simulink model "Straight_line"  (R2021a)
settings: Solver=VariableStepAuto  StartTime=0.0  StopTime=60  RelTol=1e-3  AbsTol=1e-3  EnableMultiTasking=on
values from neighbouring files (symbols this model uses):
  m = rho * V    [Tinh_I_va_m.m]
libraries: sm_lib x11, nesl_utility x10, simulink x5
settings Model: Creator=Administrator  LastModifiedBy=Administrator
settings SolverCC: AutoScaleAbsTol=off  ZeroCrossAlgorithm=Adaptive  AlgebraicLoopSolver=TrustRegion
settings DataIOCC: LimitDataPoints=on  MaxDataPoints=10000
settings OptimizationCC: LifeSpan=inf
settings DebuggingCC: IgnoredZcDiagnostic=none  AllowSymbolicDim=off  SFUnexpectedBacktrackingDiag=warning  SFNoUnconditionalDefaultTransitionDiag=warning  SFExecutionAtInitializationDiag=none  SFMachineParentedDataDiag=warning  ArithmeticOperatorsInVariantConditions=warning
settings SFSimCC: SimUseLocalCustomCode=off  CustomCodeUndefinedFunction=UseInterfaceOnly
settings RTWCC: RTWUseLocalCustomCode=off
settings CodeAppCC: StateflowObjectComments=on
settings GRTTargetCC: TargetLangStandard=C89/C90 (ANSI)
settings ConfigComp: CovMetricSettings=dw  CovSaveCumulativeToWorkspaceVar=on  CovSaveSingleToWorkspaceVar=on  CovExternalEMLEnable=off  CovSFcnEnable=off
settings SimscapeCC: SimscapeLogType=all  SimscapeLogSimulationStatistics=on  SimscapeLogDataHistory=10000

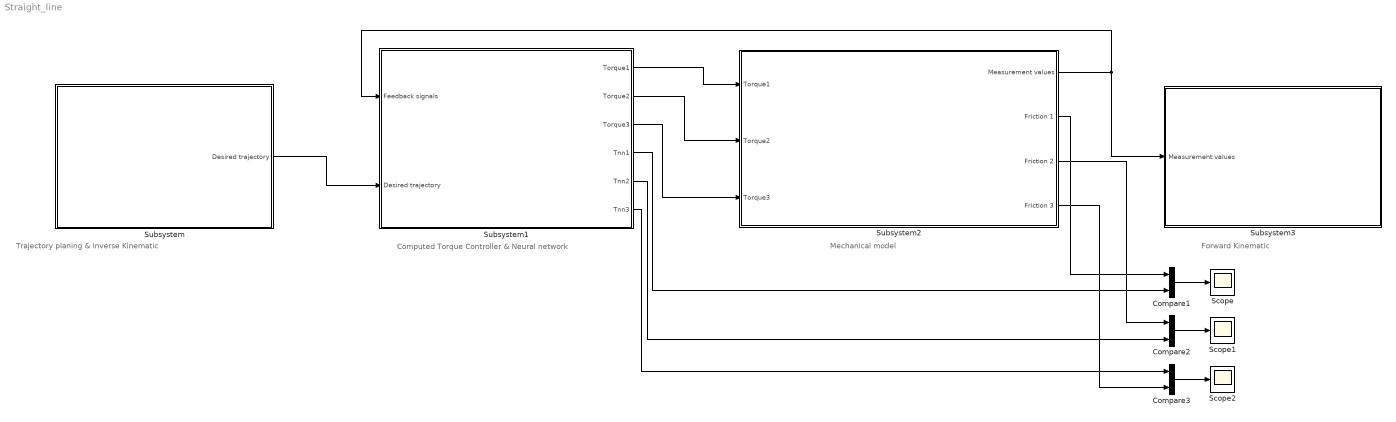
== system Straight_line ==
  note: Trajectory planing & Inverse Kinematic
  note: Computed Torque Controller
      | & Neural network
  note: Mechanical model
  note: Forward Kinematic
  Compare1 : Mux  Inputs=2
  Compare2 : Mux  Inputs=2
  Compare3 : Mux  Inputs=2
  Scope : Scope
  Scope1 : Scope
  Scope2 : Scope
  Subsystem : Subsystem
  Subsystem1 : Subsystem
  Subsystem2 : Subsystem
  Subsystem3 : Subsystem
  wires:
  Subsystem/1("Desired trajectory ") -> Subsystem1/2(Desired trajectory)
  Subsystem1/1(Torque1) -> Subsystem2/1(Torque1)
  Subsystem2/1(Measurement values) -> Subsystem1/1(Feedback signals), Subsystem3/1(Measurement values)
  Subsystem1/2(Torque2) -> Subsystem2/2(Torque2)
  Subsystem1/3(Torque3) -> Subsystem2/3(Torque3)
  Subsystem2/4(Friction 3) -> Compare3/2
  Subsystem1/6(Tnn3) -> Compare3/1
  Subsystem1/5(Tnn2) -> Compare2/2
  Subsystem2/3(Friction 2) -> Compare2/1
  Subsystem1/4(Tnn1) -> Compare1/2
  Subsystem2/2(Friction 1) -> Compare1/1
  Compare1/1 -> Scope/1
  Compare2/1 -> Scope1/1
  Compare3/1 -> Scope2/1

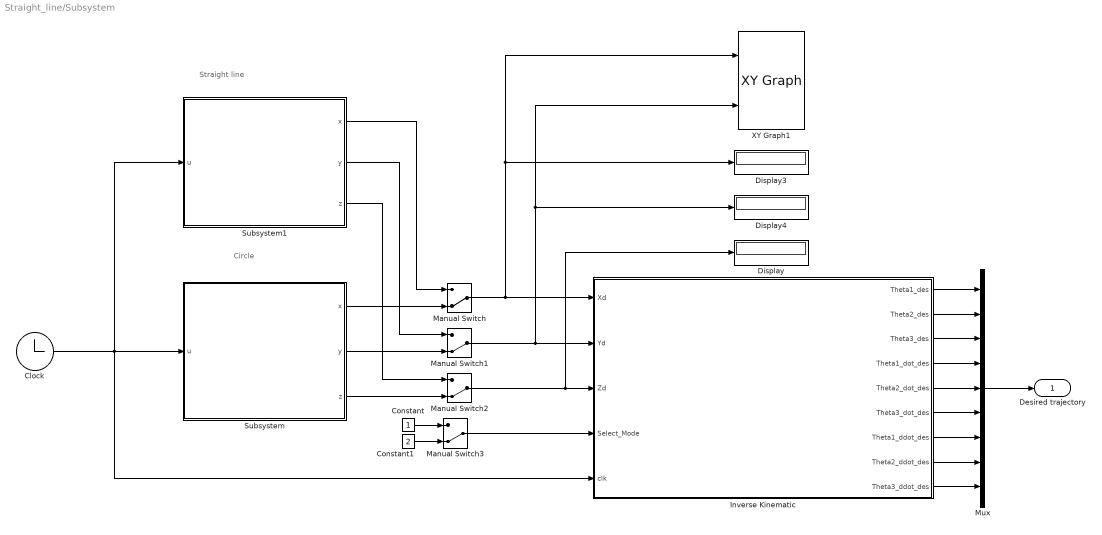
== system Straight_line/Subsystem ==
  note: Circle
  note: Straight line
  Clock : Clock
  Constant : Constant
  Constant1 : Constant  Value=2
  Display : Display
  Display3 : Display
  Display4 : Display
  Inverse Kinematic : MATLAB Function  TreatAsAtomicUnit=on
  Manual Switch{,1..3} (4 alike) : ManualSwitch  CurrentSetting=0
  Mux : Mux  Inputs=9
  Subsystem : Subsystem
  Subsystem1 : Subsystem
  XY Graph1 : simulink/Sinks/XY Graph  xmin=-3  xmax=3  ymin=-3  ymax=3  st=-1
  "Desired trajectory " : Outport
  wires:
  Clock/1 -> Subsystem1/1(u), Inverse Kinematic/5(clk), Subsystem/1(u)
  Inverse Kinematic/1(Theta1_des) -> Mux/1
  Inverse Kinematic/2(Theta2_des) -> Mux/2
  Inverse Kinematic/3(Theta3_des) -> Mux/3
  Inverse Kinematic/4(Theta1_dot_des) -> Mux/4
  Inverse Kinematic/5(Theta2_dot_des) -> Mux/5
  Inverse Kinematic/6(Theta3_dot_des) -> Mux/6
  Inverse Kinematic/7(Theta1_ddot_des) -> Mux/7
  Inverse Kinematic/8(Theta2_ddot_des) -> Mux/8
  Inverse Kinematic/9(Theta3_ddot_des) -> Mux/9
  Subsystem/1(x) -> Manual Switch/2
  Manual Switch/1 -> Inverse Kinematic/1(Xd), XY Graph1/1, Display3/1
  Manual Switch1/1 -> Inverse Kinematic/2(Yd), XY Graph1/2, Display4/1
  Subsystem/2(y) -> Manual Switch1/2
  Manual Switch2/1 -> Inverse Kinematic/3(Zd), Display/1
  Subsystem/3(z) -> Manual Switch2/2
  Mux/1 -> "Desired trajectory "/1
  Subsystem1/1(x) -> Manual Switch/1
  Subsystem1/2(y) -> Manual Switch1/1
  Subsystem1/3(z) -> Manual Switch2/1
  Manual Switch3/1 -> Inverse Kinematic/4(Select_Mode)
  Constant/1 -> Manual Switch3/1
  Constant1/1 -> Manual Switch3/2

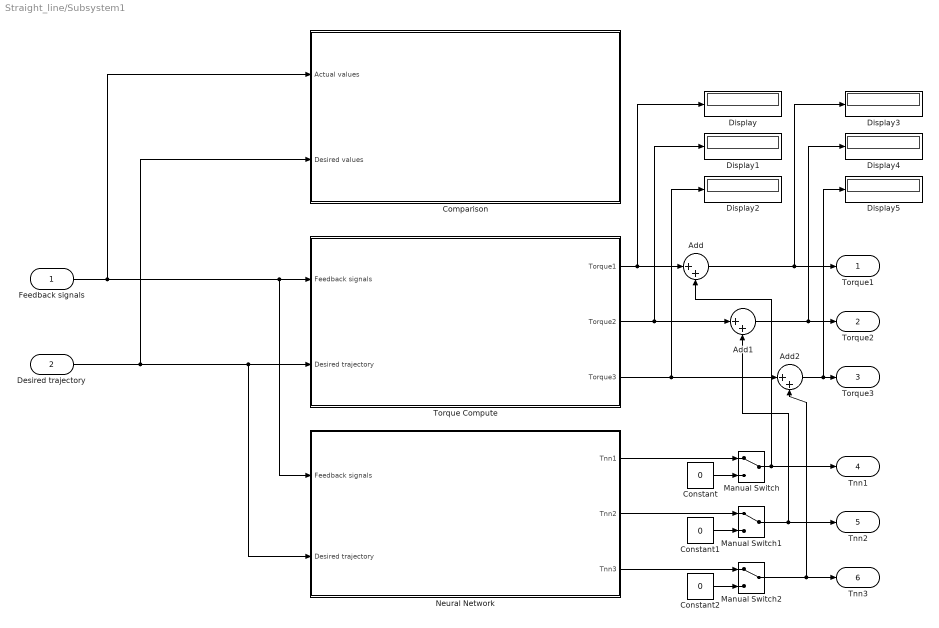
== system Straight_line/Subsystem1 ==
  Feedback signals : Inport
  Desired trajectory : Inport  Port=2
  Add : Sum  Inputs=|++
  Add1 : Sum  Inputs=|++
  Add2 : Sum  Inputs=|++
  Comparison : Subsystem
  Constant : Constant  Value=0
  Constant1 : Constant  Value=0
  Constant2 : Constant  Value=0
  Display{,1..5} (6 alike) : Display
  Manual Switch : ManualSwitch
  Manual Switch1 : ManualSwitch
  Manual Switch2 : ManualSwitch
  Neural Network : Subsystem
  Torque Compute : Subsystem
  Torque1 : Outport
  Torque2 : Outport  Port=2
  Torque3 : Outport  Port=3
  Tnn1 : Outport  Port=4
  Tnn2 : Outport  Port=5
  Tnn3 : Outport  Port=6
  wires:
  Feedback signals/1 -> Comparison/1(Actual values), Neural Network/1(Feedback signals), Torque Compute/1(Feedback signals)
  Desired trajectory/1 -> Comparison/2(Desired values), Torque Compute/2(Desired trajectory), Neural Network/2(Desired trajectory)
  Torque Compute/1(Torque1) -> Display/1, Add/1
  Torque Compute/3(Torque3) -> Display2/1, Add2/1
  Add2/1 -> Display5/1, Torque3/1
  Torque Compute/2(Torque2) -> Display1/1, Add1/1
  Add1/1 -> Display4/1, Torque2/1
  Add/1 -> Display3/1, Torque1/1
  Manual Switch/1 -> Tnn1/1, Add/2
  Constant/1 -> Manual Switch/2
  Constant2/1 -> Manual Switch2/2
  Constant1/1 -> Manual Switch1/2
  Manual Switch1/1 -> Tnn2/1, Add1/2
  Manual Switch2/1 -> Tnn3/1, Add2/2
  Neural Network/3(Tnn3) -> Manual Switch2/1
  Neural Network/2(Tnn2) -> Manual Switch1/1
  Neural Network/1(Tnn1) -> Manual Switch/1

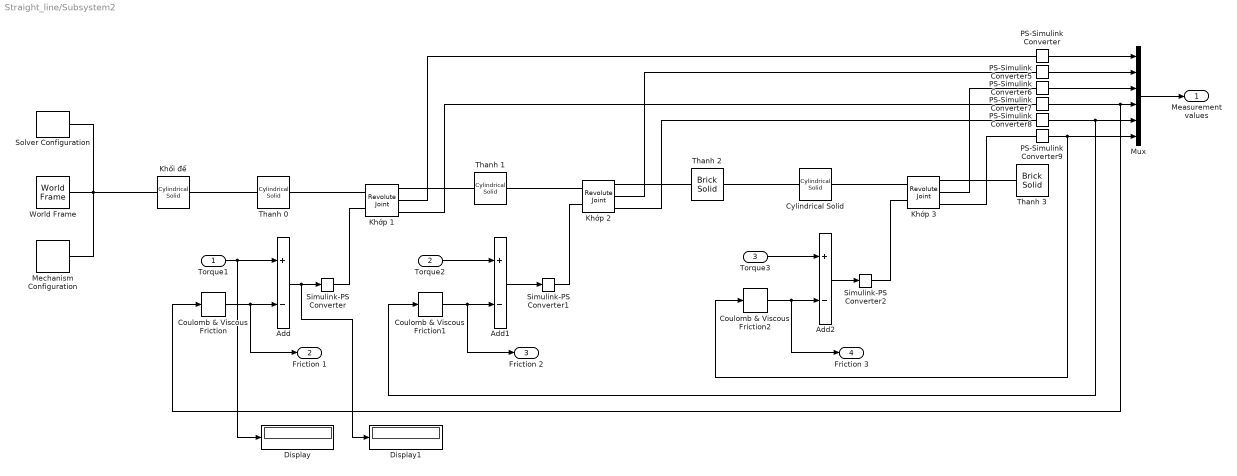
== system Straight_line/Subsystem2 ==
  Torque1 : Inport
  Torque2 : Inport  Port=2
  Torque3 : Inport  Port=3
  Add : Sum  Inputs=+-
  Add1 : Sum  Inputs=+-
  Add2 : Sum  Inputs=+-
  Coulomb & Viscous Friction : simulink/Discontinuities/Coulomb & Viscous Friction  offset=0  gain=0
  Coulomb & Viscous Friction1 : simulink/Discontinuities/Coulomb & Viscous Friction  offset=0  gain=0
  Coulomb & Viscous Friction2 : simulink/Discontinuities/Coulomb & Viscous Friction  offset=0  gain=0
  Cylindrical Solid : sm_lib/Body Elements/Cylindrical Solid  GraphicAmbientColor=[0.15 0.15 0.15 1.0]  BasedOnType=Density  CenterOfMass=[0 0 0]  CenterOfMassUnits=m  GraphicDiffuseColor=[0.8 0.4 1.0]  CylinderLength=0.5  CylinderLengthUnits=m  CylinderRadius=0.5  CylinderRadiusUnits=m  Density=900  DensityUnits=kg/m^3  DoExposeReferenceFrame=off  GraphicEmissiveColor=[0.0 0.0 0.0 1.0]  ExportEntireGeometry=off  SerializedFrames=<Frames><Frame><Id>Frame1</Id><Value><Name>F1</Name><Origin><Source>GeometricFeature</Source><FeatureName>top surface</FeatureName></Origin><PrimaryAxis><DefinedDirection>+Z</DefinedDirection><Source>ReferenceFrame</Source><SourceDirection>+Z</SourceDirection><FeatureName></FeatureName></PrimaryAxis><SecondaryAxis><DefinedDirection>+X</DefinedDirection><Source>ReferenceFrame</Source><SourceDirection>+X</SourceDirection><FeatureName></FeatureName></SecondaryAxis></Value></Frame><Frame><Id>Frame2</Id><Value><Name>F2</Name><Origin><Source>GeometricFeature</Source><FeatureName>bottom surface</FeatureName></Origin><PrimaryAxis><DefinedDirection>+Z</DefinedDirection><Source>ReferenceFrame</Source><SourceDirection>+Z</SourceDirection><FeatureName></FeatureName></PrimaryAxis><SecondaryAxis><DefinedDirection>+X</DefinedDirection><Source>ReferenceFrame</Source><SourceDirection>+X</SourceDirection><FeatureName></FeatureName></SecondaryAxis></Value></Frame></Frames>  MarkerShape=Sphere  MarkerSize=10  GraphicType=FromGeometry  InertiaType=CalculateFromGeometry  Mass=1  MassUnits=kg  MomentsOfInertia=[1 1 1]  MomentsOfInertiaUnits=kg*m^2  GraphicOpacity=1.0  ProductsOfInertia=[0 0 0]  ProductsOfInertiaUnits=kg*m^2  GraphicShininess=75  GraphicSpecularColor=[0.5 0.5 0.5 1.0]  GraphicVisPropType=SimpleVisualProperties
  Display : Display
  Display1 : Display
  Khối đế : sm_lib/Body Elements/Cylindrical Solid  GraphicAmbientColor=[0.15 0.15 0.15 1.0]  BasedOnType=Density  CenterOfMass=[0 0 0]  CenterOfMassUnits=m  GraphicDiffuseColor=[0.2 1.0 0.2]  CylinderLength=8  CylinderLengthUnits=m  CylinderRadius=3  CylinderRadiusUnits=m  Density=900  DensityUnits=kg/m^3  DoExposeReferenceFrame=on  GraphicEmissiveColor=[0.0 0.0 0.0 1.0]  ExportEntireGeometry=off  SerializedFrames=<Frames><Frame><Id>Frame1</Id><Value><Name>Top</Name><Origin><Source>GeometricFeature</Source><FeatureName>top surface</FeatureName></Origin><PrimaryAxis><DefinedDirection>+Z</DefinedDirection><Source>ReferenceFrame</Source><SourceDirection>+Z</SourceDirection><FeatureName></FeatureName></PrimaryAxis><SecondaryAxis><DefinedDirection>+X</DefinedDirection><Source>ReferenceFrame</Source><SourceDirection>+X</SourceDirection><FeatureName></FeatureName></SecondaryAxis></Value></Frame></Frames>  MarkerShape=Sphere  MarkerSize=10  GraphicType=FromGeometry  InertiaType=CalculateFromGeometry  Mass=1  MassUnits=kg  MomentsOfInertia=[1 1 1]  MomentsOfInertiaUnits=kg*m^2  GraphicOpacity=1.0  ProductsOfInertia=[0 0 0]  ProductsOfInertiaUnits=kg*m^2  GraphicShininess=75  GraphicSpecularColor=[0.5 0.5 0.5 1.0]  GraphicVisPropType=SimpleVisualProperties
  Khớp 1 : sm_lib/Joints/Revolute Joint  JointMode=Normal  SenseConstraintForce=off  SenseConstraintForceX=off  SenseConstraintForceY=off  SenseConstraintForceZ=off  SenseConstraintTorque=off  SenseConstraintTorqueX=off  SenseConstraintTorqueY=off  SenseConstraintTorqueZ=off  SenseTotalForce=off  SenseTotalForceX=off  SenseTotalForceY=off  SenseTotalForceZ=off  SenseTotalTorque=off  SenseTotalTorqueX=off  SenseTotalTorqueY=off  SenseTotalTorqueZ=off  CompositeWrenchDir=FollowerOnBase  CompositeWrenchFrame=BaseFrame  EquilibriumPosition=0  EquilibriumPositionUnits=deg  SpringStiffness=0  SpringStiffnessUnits=N*m/deg  DampingCoefficient=0  DampingCoefficientUnits=N*m/(deg/s)  TorqueActuationMode=InputTorque  MotionActuationMode=ComputedMotion  SensePosition=on  SenseVelocity=on  SenseAcceleration=off  SenseTorqueForce=off  SenseLowerLimitTorqueForce=off  SenseUpperLimitTorqueForce=off  LowerLimitSpecify=off  LowerLimitBound=-90  LowerLimitBoundUnits=deg  LowerLimitStiffness=1e4  LowerLimitStiffnessUnits=N*m/deg  LowerLimitDamping=10  LowerLimitDampingUnits=N*m/(deg/s)  LowerLimitTransitionRegionWidth=0.1  LowerLimitTransitionRegionWidthUnits=deg  UpperLimitSpecify=off  UpperLimitBound=90  UpperLimitBoundUnits=deg  UpperLimitStiffness=1e4  UpperLimitStiffnessUnits=N*m/deg  UpperLimitDamping=10  UpperLimitDampingUnits=N*m/(deg/s)  UpperLimitTransitionRegionWidth=0.1  UpperLimitTransitionRegionWidthUnits=deg  PositionTargetSpecify=off  PositionTargetPriority=High  PositionTargetValue=0  PositionTargetValueUnits=deg  VelocityTargetSpecify=off  VelocityTargetPriority=High  VelocityTargetValue=0  VelocityTargetValueUnits=deg/s
  Khớp 2 : sm_lib/Joints/Revolute Joint  JointMode=Normal  SenseConstraintForce=off  SenseConstraintForceX=off  SenseConstraintForceY=off  SenseConstraintForceZ=off  SenseConstraintTorque=off  SenseConstraintTorqueX=off  SenseConstraintTorqueY=off  SenseConstraintTorqueZ=off  SenseTotalForce=off  SenseTotalForceX=off  SenseTotalForceY=off  SenseTotalForceZ=off  SenseTotalTorque=off  SenseTotalTorqueX=off  SenseTotalTorqueY=off  SenseTotalTorqueZ=off  CompositeWrenchDir=FollowerOnBase  CompositeWrenchFrame=BaseFrame  EquilibriumPosition=0  EquilibriumPositionUnits=deg  SpringStiffness=0  SpringStiffnessUnits=N*m/deg  DampingCoefficient=0  DampingCoefficientUnits=N*m/(deg/s)  TorqueActuationMode=InputTorque  MotionActuationMode=ComputedMotion  SensePosition=on  SenseVelocity=on  SenseAcceleration=off  SenseTorqueForce=off  SenseLowerLimitTorqueForce=off  SenseUpperLimitTorqueForce=off  LowerLimitSpecify=off  LowerLimitBound=-90  LowerLimitBoundUnits=deg  LowerLimitStiffness=1e4  LowerLimitStiffnessUnits=N*m/deg  LowerLimitDamping=10  LowerLimitDampingUnits=N*m/(deg/s)  LowerLimitTransitionRegionWidth=0.1  LowerLimitTransitionRegionWidthUnits=deg  UpperLimitSpecify=off  UpperLimitBound=90  UpperLimitBoundUnits=deg  UpperLimitStiffness=1e4  UpperLimitStiffnessUnits=N*m/deg  UpperLimitDamping=10  UpperLimitDampingUnits=N*m/(deg/s)  UpperLimitTransitionRegionWidth=0.1  UpperLimitTransitionRegionWidthUnits=deg  PositionTargetSpecify=off  PositionTargetPriority=High  PositionTargetValue=0  PositionTargetValueUnits=deg  VelocityTargetSpecify=off  VelocityTargetPriority=High  VelocityTargetValue=0  VelocityTargetValueUnits=deg/s
  Khớp 3 : sm_lib/Joints/Revolute Joint  JointMode=Normal  SenseConstraintForce=off  SenseConstraintForceX=off  SenseConstraintForceY=off  SenseConstraintForceZ=off  SenseConstraintTorque=off  SenseConstraintTorqueX=off  SenseConstraintTorqueY=off  SenseConstraintTorqueZ=off  SenseTotalForce=off  SenseTotalForceX=off  SenseTotalForceY=off  SenseTotalForceZ=off  SenseTotalTorque=off  SenseTotalTorqueX=off  SenseTotalTorqueY=off  SenseTotalTorqueZ=off  CompositeWrenchDir=FollowerOnBase  CompositeWrenchFrame=BaseFrame  EquilibriumPosition=0  EquilibriumPositionUnits=deg  SpringStiffness=0  SpringStiffnessUnits=N*m/deg  DampingCoefficient=0  DampingCoefficientUnits=N*m/(deg/s)  TorqueActuationMode=InputTorque  MotionActuationMode=ComputedMotion  SensePosition=on  SenseVelocity=on  SenseAcceleration=off  SenseTorqueForce=off  SenseLowerLimitTorqueForce=off  SenseUpperLimitTorqueForce=off  LowerLimitSpecify=off  LowerLimitBound=-90  LowerLimitBoundUnits=deg  LowerLimitStiffness=1e4  LowerLimitStiffnessUnits=N*m/deg  LowerLimitDamping=10  LowerLimitDampingUnits=N*m/(deg/s)  LowerLimitTransitionRegionWidth=0.1  LowerLimitTransitionRegionWidthUnits=deg  UpperLimitSpecify=off  UpperLimitBound=90  UpperLimitBoundUnits=deg  UpperLimitStiffness=1e4  UpperLimitStiffnessUnits=N*m/deg  UpperLimitDamping=10  UpperLimitDampingUnits=N*m/(deg/s)  UpperLimitTransitionRegionWidth=0.1  UpperLimitTransitionRegionWidthUnits=deg  PositionTargetSpecify=off  PositionTargetPriority=High  PositionTargetValue=0  PositionTargetValueUnits=deg  VelocityTargetSpecify=off  VelocityTargetPriority=High  VelocityTargetValue=0  VelocityTargetValueUnits=deg/s
  Mechanism Configuration : sm_lib/Utilities/Mechanism Configuration  UniformGravity=Constant  GravityVector=[0 0 -9.80665]  GravityVectorUnits=m/s^2  GravityUnits=m/s^2  LinearizationDelta=0.001  JointModeTransitionNonlinearIterations=2
  Mux : Mux  Inputs=6
  PS-Simulink Converter{,5..9} (6 alike) : nesl_utility/PS-Simulink Converter  PhysicalDomain=network_engine_domain  SubClassName=ps_output  LeftPortType=input  RightPortType=output  PseudoPeriodic=off  Frequencies=[]  Unit=inherit  AffineConversion=off
      settings: SourceProductBaseCode=PW,SS
  Simulink-PS Converter : nesl_utility/Simulink-PS Converter  PhysicalDomain=network_engine_domain  SubClassName=ps_input  LeftPortType=input  RightPortType=output  PseudoPeriodic=off  Frequencies=[]  NoiseDistribution=none  NoiseParameters=[]  Unit=1  AffineConversion=off  FilteringAndDerivatives=provide  SimscapeFilterOrder=1  InputFilterTimeConstant=0.001  UdotUserProvided=0
      settings: SourceProductBaseCode=PW,SS
  Simulink-PS Converter1 : nesl_utility/Simulink-PS Converter  PhysicalDomain=network_engine_domain  SubClassName=ps_input  LeftPortType=input  RightPortType=output  PseudoPeriodic=off  Frequencies=[]  NoiseDistribution=none  NoiseParameters=[]  Unit=1  AffineConversion=off  FilteringAndDerivatives=provide  SimscapeFilterOrder=1  InputFilterTimeConstant=0.001  UdotUserProvided=0
      settings: SourceProductBaseCode=PW,SS
  Simulink-PS Converter2 : nesl_utility/Simulink-PS Converter  PhysicalDomain=network_engine_domain  SubClassName=ps_input  LeftPortType=input  RightPortType=output  PseudoPeriodic=off  Frequencies=[]  NoiseDistribution=none  NoiseParameters=[]  Unit=1  AffineConversion=off  FilteringAndDerivatives=provide  SimscapeFilterOrder=1  InputFilterTimeConstant=0.001  UdotUserProvided=0
      settings: SourceProductBaseCode=PW,SS
  Solver Configuration : nesl_utility/Solver Configuration  PhysicalDomain=network_engine_domain  SubClassName=solver  LeftPortType=input  RightPortType=generic  Tones=[]  Harmonics=[]  SimulateNoise=off  Profile=off  UseLocalSampling=off  EnableSwitchedLinearOptims=on  FrequencyDomain=off  UseCCode=off  RelTol=0.001  AbsTol=1e-06  MinStep=1e-09  ToWorkspace=off  RevertToSquareIcSolve=off  NumHomotopyIterations=100  PhasorMode=off  PhasorModeNumHarmonics=1  DoDC=off  ResidualTolerance=1e-09  UseLocalSolver=off  LocalSolverChoice=NE_BACKWARD_EULER_ADVANCER  LocalSolverSampleTime=0.001  DoFixedCost=off  MaxNonlinIter=3  MaxModeIter=2  ComputeImpulses=off  ImpulseIterations=2  LinearAlgebra=Sparse  EquationFormulation=NE_TIME_EF  DelaysMemoryBudget=1024  AutomaticFiltering=on  FilteringTimeConstant=0.001  PartitionStorageMethod=AS_NEEDED  PartitionMemoryBudget=1024  PartitionMethod=FAST
      settings: SourceProductBaseCode=PW,SS
  Thanh 0 : sm_lib/Body Elements/Cylindrical Solid  GraphicAmbientColor=[0.15 0.15 0.15 1.0]  BasedOnType=Density  CenterOfMass=[0 0 0]  CenterOfMassUnits=m  GraphicDiffuseColor=[1.0 1.0 0.0]  CylinderLength=5  CylinderLengthUnits=m  CylinderRadius=2  CylinderRadiusUnits=m  Density=900  DensityUnits=kg/m^3  DoExposeReferenceFrame=off  GraphicEmissiveColor=[0.0 0.0 0.0 1.0]  ExportEntireGeometry=off  SerializedFrames=<Frames><Frame><Id>Frame1</Id><Value><Name>Bottom</Name><Origin><Source>GeometricFeature</Source><FeatureName>bottom surface</FeatureName></Origin><PrimaryAxis><DefinedDirection>+Z</DefinedDirection><Source>ReferenceFrame</Source><SourceDirection>+Z</SourceDirection><FeatureName></FeatureName></PrimaryAxis><SecondaryAxis><DefinedDirection>+X</DefinedDirection><Source>ReferenceFrame</Source><SourceDirection>+X</SourceDirection><FeatureName></FeatureName></SecondaryAxis></Value></Frame><Frame><Id>Frame2</Id><Value><Name>Top</Name><Origin><Source>GeometricFeature</Source><FeatureName>top surface</FeatureName></Origin><PrimaryAxis><DefinedDirection>+Z</DefinedDirection><Source>ReferenceFrame</Source><SourceDirection>+Z</SourceDirection><FeatureName></FeatureName></PrimaryAxis><SecondaryAxis><DefinedDirection>+X</DefinedDirection><Source>ReferenceFrame</Source><SourceDirection>+X</SourceDirection><FeatureName></FeatureName></SecondaryAxis></Value></Frame></Frames>  MarkerShape=Sphere  MarkerSize=10  GraphicType=FromGeometry  InertiaType=CalculateFromGeometry  Mass=1  MassUnits=kg  MomentsOfInertia=[1 1 1]  MomentsOfInertiaUnits=kg*m^2  GraphicOpacity=1.0  ProductsOfInertia=[0 0 0]  ProductsOfInertiaUnits=kg*m^2  GraphicShininess=75  GraphicSpecularColor=[0.5 0.5 0.5 1.0]  GraphicVisPropType=SimpleVisualProperties
  Thanh 1 : sm_lib/Body Elements/Cylindrical Solid  GraphicAmbientColor=[0.15 0.15 0.15 1.0]  BasedOnType=Density  CenterOfMass=[0 0 0]  CenterOfMassUnits=m  GraphicDiffuseColor=[0.2 1.0 0.8]  CylinderLength=7  CylinderLengthUnits=m  CylinderRadius=2  CylinderRadiusUnits=m  Density=900  DensityUnits=kg/m^3  DoExposeReferenceFrame=off  GraphicEmissiveColor=[0.0 0.0 0.0 1.0]  ExportEntireGeometry=off  SerializedFrames=<Frames><Frame><Id>Frame1</Id><Value><Name>Left</Name><Origin><Source>GeometricFeature</Source><FeatureName>top surface</FeatureName></Origin><PrimaryAxis><DefinedDirection>+Z</DefinedDirection><Source>ReferenceFrame</Source><SourceDirection>+Z</SourceDirection><FeatureName></FeatureName></PrimaryAxis><SecondaryAxis><DefinedDirection>+X</DefinedDirection><Source>ReferenceFrame</Source><SourceDirection>+X</SourceDirection><FeatureName></FeatureName></SecondaryAxis></Value></Frame><Frame><Id>Frame2</Id><Value><Name>Mid</Name><Origin><Source>CenterOfMassFrame</Source><FeatureName></FeatureName></Origin><PrimaryAxis><DefinedDirection>+Y</DefinedDirection><Source>ReferenceFrame</Source><SourceDirection>+Z</SourceDirection><FeatureName></FeatureName></PrimaryAxis><SecondaryAxis><DefinedDirection>+X</DefinedDirection><Source>ReferenceFrame</Source><SourceDirection>+X</SourceDirection><FeatureName></FeatureName></SecondaryAxis></Value></Frame></Frames>  MarkerShape=Sphere  MarkerSize=10  GraphicType=FromGeometry  InertiaType=CalculateFromGeometry  Mass=1  MassUnits=kg  MomentsOfInertia=[1 1 1]  MomentsOfInertiaUnits=kg*m^2  GraphicOpacity=1.0  ProductsOfInertia=[0 0 0]  ProductsOfInertiaUnits=kg*m^2  GraphicShininess=75  GraphicSpecularColor=[0.5 0.5 0.5 1.0]  GraphicVisPropType=SimpleVisualProperties
  Thanh 2 : sm_lib/Body Elements/Brick Solid  GraphicAmbientColor=[0.15 0.15 0.15 1.0]  BasedOnType=Density  BrickDimensions=[3 1 11]  BrickDimensionUnits=m  CenterOfMass=[0 0 0]  CenterOfMassUnits=m  GraphicDiffuseColor=[1.0 0.6 0.6]  Density=9000  DensityUnits=kg/m^3  DoExposeReferenceFrame=off  GraphicEmissiveColor=[0.0 0.0 0.0 1.0]  ExportEntireGeometry=off  SerializedFrames=<Frames><Frame><Id>Frame1</Id><Value><Name>F1</Name><Origin><Source>GeometricFeature</Source><FeatureName>-z surface</FeatureName></Origin><PrimaryAxis><DefinedDirection>+X</DefinedDirection><Source>ReferenceFrame</Source><SourceDirection>+Z</SourceDirection><FeatureName></FeatureName></PrimaryAxis><SecondaryAxis><DefinedDirection>+Y</DefinedDirection><Source>ReferenceFrame</Source><SourceDirection>+X</SourceDirection><FeatureName></FeatureName></SecondaryAxis></Value></Frame><Frame><Id>Frame2</Id><Value><Name>F2</Name><Origin><Source>GeometricFeature</Source><FeatureName>+z surface</FeatureName></Origin><PrimaryAxis><DefinedDirection>+X</DefinedDirection><Source>ReferenceFrame</Source><SourceDirection>+Z</SourceDirection><FeatureName></FeatureName></PrimaryAxis><SecondaryAxis><DefinedDirection>+Y</DefinedDirection><Source>ReferenceFrame</Source><SourceDirection>+X</SourceDirection><FeatureName></FeatureName></SecondaryAxis></Value></Frame></Frames>  MarkerShape=Sphere  MarkerSize=10  GraphicType=FromGeometry  InertiaType=CalculateFromGeometry  Mass=1  MassUnits=kg  MomentsOfInertia=[1 1 1]  MomentsOfInertiaUnits=kg*m^2  GraphicOpacity=1.0  ProductsOfInertia=[0 0 0]  ProductsOfInertiaUnits=kg*m^2  GraphicShininess=75  GraphicSpecularColor=[0.5 0.5 0.5 1.0]  GraphicVisPropType=SimpleVisualProperties
  Thanh 3 : sm_lib/Body Elements/Brick Solid  GraphicAmbientColor=[0.15 0.15 0.15 1.0]  BasedOnType=Density  BrickDimensions=[2 0.5 7]  BrickDimensionUnits=m  CenterOfMass=[0 0 0]  CenterOfMassUnits=m  GraphicDiffuseColor=[0.2 1.0 0.8]  Density=9000  DensityUnits=kg/m^3  DoExposeReferenceFrame=off  GraphicEmissiveColor=[0.0 0.0 0.0 1.0]  ExportEntireGeometry=off  SerializedFrames=<Frames><Frame><Id>Frame1</Id><Value><Name>F1</Name><Origin><Source>GeometricFeature</Source><FeatureName>+z surface</FeatureName></Origin><PrimaryAxis><DefinedDirection>+X</DefinedDirection><Source>ReferenceFrame</Source><SourceDirection>+Z</SourceDirection><FeatureName></FeatureName></PrimaryAxis><SecondaryAxis><DefinedDirection>+Y</DefinedDirection><Source>ReferenceFrame</Source><SourceDirection>+X</SourceDirection><FeatureName></FeatureName></SecondaryAxis></Value></Frame><Frame><Id>Frame2</Id><Value><Name>F2</Name><Origin><Source>GeometricFeature</Source><FeatureName>-z surface</FeatureName></Origin><PrimaryAxis><DefinedDirection>+X</DefinedDirection><Source>ReferenceFrame</Source><SourceDirection>+Z</SourceDirection><FeatureName></FeatureName></PrimaryAxis><SecondaryAxis><DefinedDirection>+Y</DefinedDirection><Source>ReferenceFrame</Source><SourceDirection>+X</SourceDirection><FeatureName></FeatureName></SecondaryAxis></Value></Frame></Frames>  MarkerShape=Sphere  MarkerSize=10  GraphicType=FromGeometry  InertiaType=CalculateFromGeometry  Mass=1  MassUnits=kg  MomentsOfInertia=[1 1 1]  MomentsOfInertiaUnits=kg*m^2  GraphicOpacity=1.0  ProductsOfInertia=[0 0 0]  ProductsOfInertiaUnits=kg*m^2  GraphicShininess=75  GraphicSpecularColor=[0.5 0.5 0.5 1.0]  GraphicVisPropType=SimpleVisualProperties
  World Frame : sm_lib/Frames and Transforms/World Frame
  Measurement values : Outport
  Friction 1 : Outport  Port=2
  Friction 2 : Outport  Port=3
  Friction 3 : Outport  Port=4
  wires:
  PS-Simulink Converter/1 -> Mux/1
  PS-Simulink Converter5/1 -> Mux/2
  PS-Simulink Converter6/1 -> Mux/3
  PS-Simulink Converter7/1 -> Coulomb & Viscous Friction/1, Mux/4
  PS-Simulink Converter8/1 -> Coulomb & Viscous Friction1/1, Mux/5
  PS-Simulink Converter9/1 -> Coulomb & Viscous Friction2/1, Mux/6
  Mux/1 -> Measurement values/1
  Torque1/1 -> Display/1, Add/1
  Coulomb & Viscous Friction/1 -> Friction 1/1, Add/2
  Add/1 -> Display1/1, Simulink-PS Converter/1
  Coulomb & Viscous Friction1/1 -> Friction 2/1, Add1/2
  Torque2/1 -> Add1/1
  Add1/1 -> Simulink-PS Converter1/1
  Torque3/1 -> Add2/1
  Coulomb & Viscous Friction2/1 -> Friction 3/1, Add2/2
  Add2/1 -> Simulink-PS Converter2/1
  connections:
  Khớp 3/LConn1 -- Cylindrical Solid/RConn1
  Thanh 0/RConn1 -- Khớp 1/LConn1
  World Frame/RConn1 -- Mechanism Configuration/RConn1 -- Khối đế/RConn1 -- Solver Configuration/RConn1
  Khớp 2/LConn1 -- Thanh 1/LConn1
  Khớp 2/RConn1 -- Thanh 2/RConn1
  Khối đế/LConn1 -- Thanh 0/LConn1
  Thanh 3/LConn1 -- Khớp 3/RConn1
  Thanh 2/LConn1 -- Cylindrical Solid/LConn1
  Khớp 1/RConn1 -- Thanh 1/RConn1
  Khớp 1/RConn2 -- PS-Simulink Converter/LConn1
  Khớp 1/RConn3 -- PS-Simulink Converter7/LConn1
  Khớp 2/RConn2 -- PS-Simulink Converter5/LConn1
  Khớp 2/RConn3 -- PS-Simulink Converter8/LConn1
  Khớp 3/RConn2 -- PS-Simulink Converter6/LConn1
  Khớp 3/RConn3 -- PS-Simulink Converter9/LConn1
  Simulink-PS Converter/RConn1 -- Khớp 1/LConn2
  Simulink-PS Converter1/RConn1 -- Khớp 2/LConn2
  Simulink-PS Converter2/RConn1 -- Khớp 3/LConn2

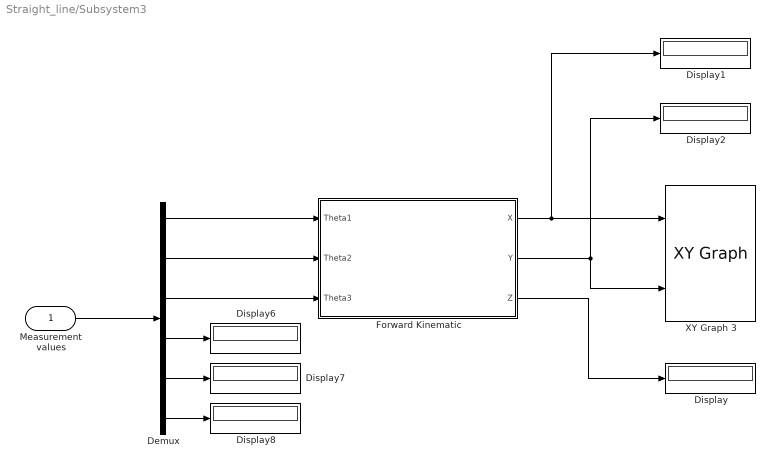
== system Straight_line/Subsystem3 ==
  Measurement values : Inport
  Demux : Demux  Outputs=6
  Display{,1..2,6..8} (6 alike) : Display
  Forward Kinematic : MATLAB Function  TreatAsAtomicUnit=on
  XY Graph 3 : simulink/Sinks/XY Graph  xmin=-3  xmax=3  ymin=-3  ymax=3  st=-1
  wires:
  Forward Kinematic/3(Z) -> Display/1
  Forward Kinematic/1(X) -> Display1/1, XY Graph 3/1
  Forward Kinematic/2(Y) -> Display2/1, XY Graph 3/2
  Demux/1 -> Forward Kinematic/1(Theta1)
  Demux/2 -> Forward Kinematic/2(Theta2)
  Demux/3 -> Forward Kinematic/3(Theta3)
  Measurement values/1 -> Demux/1
  Demux/4 -> Display6/1
  Demux/6 -> Display8/1
  Demux/5 -> Display7/1

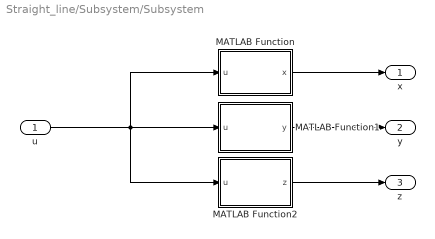
== system Straight_line/Subsystem/Subsystem ==
  u : Inport
  MATLAB Function : MATLAB Function  TreatAsAtomicUnit=on
  MATLAB Function1 : MATLAB Function  TreatAsAtomicUnit=on
  MATLAB Function2 : MATLAB Function  TreatAsAtomicUnit=on
  x : Outport
  y : Outport  Port=2
  z : Outport  Port=3
  wires:
  u/1 -> MATLAB Function2/1(u), MATLAB Function/1(u), MATLAB Function1/1(u)
  MATLAB Function/1(x) -> x/1
  MATLAB Function1/1(y) -> y/1
  MATLAB Function2/1(z) -> z/1

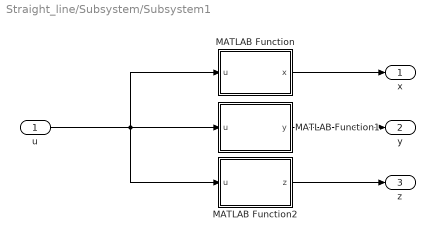
== system Straight_line/Subsystem/Subsystem1 ==
  u : Inport
  MATLAB Function : MATLAB Function  TreatAsAtomicUnit=on
  MATLAB Function1 : MATLAB Function  TreatAsAtomicUnit=on
  MATLAB Function2 : MATLAB Function  TreatAsAtomicUnit=on
  x : Outport
  y : Outport  Port=2
  z : Outport  Port=3
  wires:
  MATLAB Function1/1(y) -> y/1
  MATLAB Function2/1(z) -> z/1
  u/1 -> MATLAB Function2/1(u), MATLAB Function/1(u), MATLAB Function1/1(u)
  MATLAB Function/1(x) -> x/1

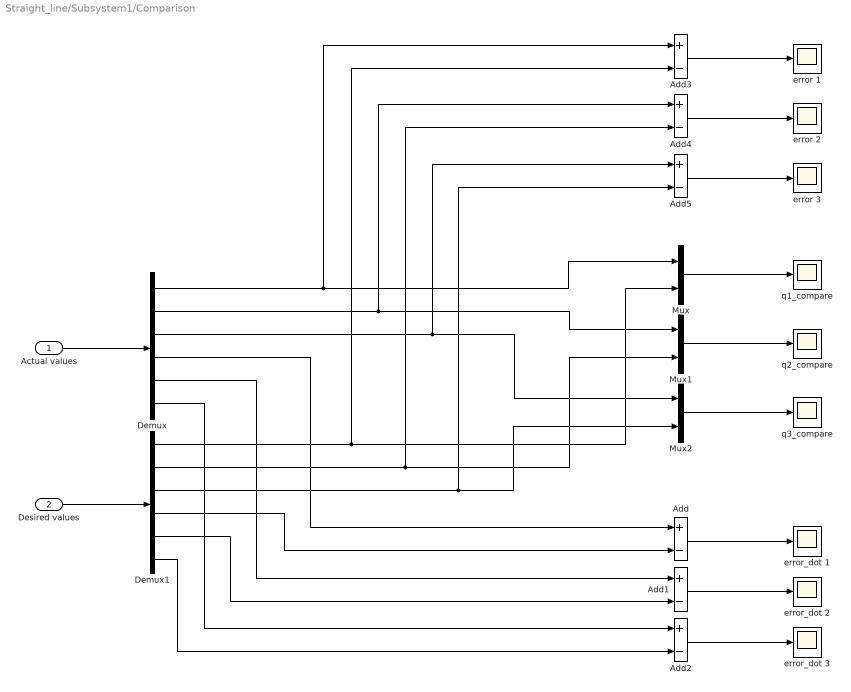
== system Straight_line/Subsystem1/Comparison ==
  Actual values : Inport
  Desired values : Inport  Port=2
  Add{,1..5} (6 alike) : Sum  Inputs=+-
  Demux : Demux  Outputs=6
  Demux1 : Demux  Outputs=6
  Mux : Mux  Inputs=2
  Mux1 : Mux  Inputs=2
  Mux2 : Mux  Inputs=2
  error 1 : Scope
  error 2 : Scope
  error 3 : Scope
  error_dot 1 : Scope
  error_dot 2 : Scope
  error_dot 3 : Scope
  q1_compare : Scope
  q2_compare : Scope
  q3_compare : Scope
  wires:
  Actual values/1 -> Demux/1
  Desired values/1 -> Demux1/1
  Mux/1 -> q1_compare/1
  Mux1/1 -> q2_compare/1
  Mux2/1 -> q3_compare/1
  Demux1/1 -> Add3/2, Mux/2
  Demux1/2 -> Add4/2, Mux1/2
  Demux1/3 -> Add5/2, Mux2/2
  Demux/1 -> Add3/1, Mux/1
  Demux/2 -> Add4/1, Mux1/1
  Demux/3 -> Add5/1, Mux2/1
  Demux/4 -> Add/1
  Demux1/4 -> Add/2
  Demux/5 -> Add1/1
  Demux1/5 -> Add1/2
  Demux/6 -> Add2/1
  Demux1/6 -> Add2/2
  Add3/1 -> error 1/1
  Add4/1 -> error 2/1
  Add5/1 -> error 3/1
  Add2/1 -> error_dot 3/1
  Add1/1 -> error_dot 2/1
  Add/1 -> error_dot 1/1

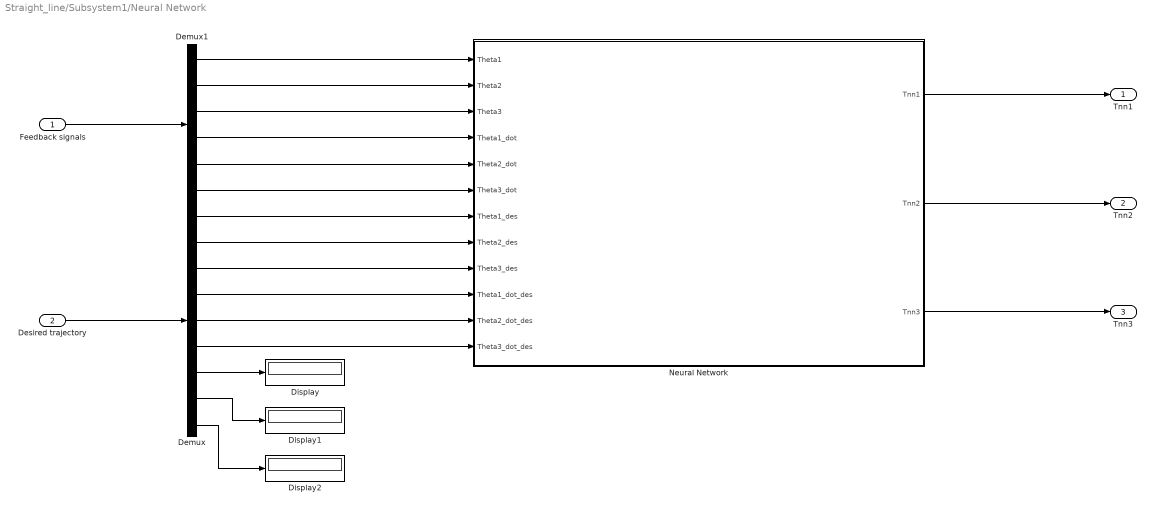
== system Straight_line/Subsystem1/Neural Network ==
  Feedback signals : Inport
  Desired trajectory : Inport  Port=2
  Demux : Demux  Outputs=9
  Demux1 : Demux  Outputs=6
  Display : Display
  Display1 : Display
  Display2 : Display
  Neural Network : MATLAB Function  TreatAsAtomicUnit=on  SystemSampleTime=0.001
  Tnn1 : Outport
  Tnn2 : Outport  Port=2
  Tnn3 : Outport  Port=3
  wires:
  Demux1/1 -> Neural Network/1(Theta1)
  Demux1/2 -> Neural Network/2(Theta2)
  Demux1/3 -> Neural Network/3(Theta3)
  Demux1/4 -> Neural Network/4(Theta1_dot)
  Demux1/5 -> Neural Network/5(Theta2_dot)
  Demux1/6 -> Neural Network/6(Theta3_dot)
  Demux/1 -> Neural Network/7(Theta1_des)
  Demux/2 -> Neural Network/8(Theta2_des)
  Demux/3 -> Neural Network/9(Theta3_des)
  Demux/4 -> Neural Network/10(Theta1_dot_des)
  Demux/5 -> Neural Network/11(Theta2_dot_des)
  Demux/6 -> Neural Network/12(Theta3_dot_des)
  Feedback signals/1 -> Demux1/1
  Desired trajectory/1 -> Demux/1
  Neural Network/1(Tnn1) -> Tnn1/1
  Neural Network/2(Tnn2) -> Tnn2/1
  Neural Network/3(Tnn3) -> Tnn3/1
  Demux/7 -> Display/1
  Demux/8 -> Display1/1
  Demux/9 -> Display2/1

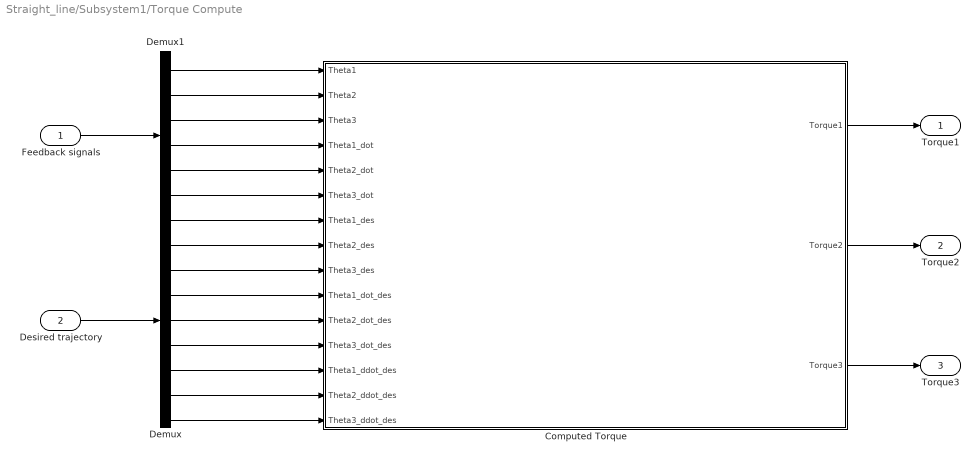
== system Straight_line/Subsystem1/Torque Compute ==
  Feedback signals : Inport
  Desired trajectory : Inport  Port=2
  Computed Torque : MATLAB Function  TreatAsAtomicUnit=on
  Demux : Demux  Outputs=9
  Demux1 : Demux  Outputs=6
  Torque1 : Outport
  Torque2 : Outport  Port=2
  Torque3 : Outport  Port=3
  wires:
  Demux/1 -> Computed Torque/7(Theta1_des)
  Demux/2 -> Computed Torque/8(Theta2_des)
  Demux/3 -> Computed Torque/9(Theta3_des)
  Demux/4 -> Computed Torque/10(Theta1_dot_des)
  Demux/5 -> Computed Torque/11(Theta2_dot_des)
  Demux/6 -> Computed Torque/12(Theta3_dot_des)
  Demux/8 -> Computed Torque/14(Theta2_ddot_des)
  Demux/7 -> Computed Torque/13(Theta1_ddot_des)
  Demux/9 -> Computed Torque/15(Theta3_ddot_des)
  Computed Torque/1(Torque1) -> Torque1/1
  Demux1/1 -> Computed Torque/1(Theta1)
  Demux1/2 -> Computed Torque/2(Theta2)
  Demux1/3 -> Computed Torque/3(Theta3)
  Demux1/4 -> Computed Torque/4(Theta1_dot)
  Demux1/5 -> Computed Torque/5(Theta2_dot)
  Demux1/6 -> Computed Torque/6(Theta3_dot)
  Feedback signals/1 -> Demux1/1
  Desired trajectory/1 -> Demux/1
  Computed Torque/2(Torque2) -> Torque2/1
  Computed Torque/3(Torque3) -> Torque3/1

== matlab function Straight_line/Subsystem/Subsystem/MATLAB Function2 ==
  data: u input; z output
function z = Ze_func(u)

    z =  -6;
    %z = -14; %chiều cao robot (đế: 8m, thanh 0: 5m, thanh 1: 1m vì nằm ngang =>vừa tầm end-effector)
end

== matlab function Straight_line/Subsystem1/Neural Network/Neural Network ==
  settings: updateMethod=DISCRETE  sampleTime=0.001
  data: Theta1 input; Tnn1 output; Theta2 input; Theta3 input; Theta1_dot input; Theta2_dot input; Theta3_dot input; Theta1_des input; Theta2_des input; Tnn2 output; Theta3_des input; Theta1_dot_des input; Theta2_dot_des input; Theta3_dot_des input; Tnn3 output
function [Tnn1, Tnn2, Tnn3] = fcn(Theta1, Theta2, Theta3, Theta1_dot, Theta2_dot, Theta3_dot, Theta1_des, Theta2_des, Theta3_des, Theta1_dot_des, Theta2_dot_des, Theta3_dot_des)
% Neural Network Controller for RRR Robot (3 DOF)
% Input: 12 inputs (Position and Velocity: Actual vs Desired for 3 joints)
% Output: 3 Torques (Tnn1, Tnn2, Tnn3)

persistent W C X S

% Khoi tao ma tran trong so ban dau
if isempty(W)
    % Tang khoi tao len mot chut de mang co tin hieu ban dau
    W = 0.1 * (2*rand(6, 10) - 1); 
    C = 0.0 * zeros(10, 3); 
    X = ones(6, 1);
    S = ones(3, 1);
end

%% 1. Input of neural network (Sai so vi tri va van toc)
% Error position
e1 = Theta1 - Theta1_des;
e2 = Theta2 - Theta2_des;
e3 = Theta3 - Theta3_des;

% Error velocity
ed1 = Theta1_dot - Theta1_dot_des;
ed2 = Theta2_dot - Theta2_dot_des;
ed3 = Theta3_dot - Theta3_dot_des;

% --- VU KHI 1: KHUECH DAI DAU VAO ---
Input_Gain = 50; 

X(1) = e1 * Input_Gain;
X(2) = e2 * Input_Gain;
X(3) = e3 * Input_Gain;
X(4) = ed1 * Input_Gain;
X(5) = ed2 * Input_Gain;
X(6) = ed3 * Input_Gain;

%X(1) = e1;
%X(2) = e2;
%X(3) = e3;
%X(4) = ed1;
%X(5) = ed2;
%X(6) = ed3;

%% 2. Sliding surface (Mat truot)
lamda1 = 6; lamda2 = 6; lamda3 = 6;

s1 = e1 + lamda1 * ed1;
s2 = e2 + lamda2 * ed2;
s3 = e3 + lamda3 * ed3;

S(1) = s1;
S(2) = s2;
S(3) = s3;
S = S .* (abs(S) > 0.002); 

%% 3. Hidden Layer Computation
H_net = zeros(10, 1);
H_out = zeros(10, 1);

% Compute H_net(j)
for j = 1:10
    for i = 1:6
        H_net(j) = H_net(j) + W(i, j) * X(i);
    end
end

% Compute H_out(j)
for j = 1:10
    Net1 = H_net(j);
    H_out(j) = (1 - exp(-Net1)) / (1 + exp(-Net1));
end

%% 4. OUTPUT LAYER (Compute Torques)
% --- KHUECH DAI DAU RA ---
% Robot nang hang chuc tan, can Torque hang tram nghin Nm
Scale_Factor = 500000; % Nhan 500,000 lan

T_net = zeros(3, 1);
for k = 1:3
    for j = 1:10
        % Tinh toan thuan tuy
        val = C(j, k) * H_out(j);
        % Nhan voi Scale Factor de ra luc thuc te
        T_net(k) = T_net(k) + val * Scale_Factor;
    end
end

%% 5. UPDATE WEIGHTS
% Learning rate (Toc do hoc)
% Vi dau ra da nhan Scale_Factor lon, nen toc do hoc phai NHO LAI
m = 0.001; 
n = 0.001; 

% Update for Output layer (C)
for j = 1:10
    for k = 1:3
        C(j, k) = C(j, k) - m * S(k) * H_out(j);
    end
end

% Update for Hidden layer (W)
for i = 1:6 
    for j = 1:10
        Delta_Wij = 0;
        for k = 1:3
            Delta_Wij = Delta_Wij + C(j, k) * S(k);
        end
        W(i, j) = W(i, j) - n * Delta_Wij * (1 - H_out(j)^2) * X(i) / 2;
    end
end

%% 6. Final Output with Saturation
% Gioi han bao hoa de tranh robot bi văng (Safety)
T_limit = 3000000; % 3 Trieu Nm

Tnn1 = max(min(T_net(1), T_limit), -T_limit);
Tnn2 = max(min(T_net(2), T_limit), -T_limit);
Tnn3 = max(min(T_net(3), T_limit), -T_limit);

end

== matlab function Straight_line/Subsystem/Subsystem1/MATLAB Function ==
  data: u input; x output
function x = Xe_func(u)
% Xe_func: Quy dao duong thang tu x = -2 den x = 2
% Su dung quy dao Cosine de van toc bat dau va ket thuc bang 0 

    % Thoi gian du kien de di tu -2 den 2 
    
    RunTime = 25; 
    
    Start_Point = -2;
    End_Point = 2;
    
    if u <= RunTime
        % u = 0 -> cos(0)=1 -> x = Start
        % u = RunTime -> cos(pi)=-1 -> x = End
        
        Center = (Start_Point + End_Point) / 2;
        Amplitude = (Start_Point - End_Point) / 2;
        
        x = Center + Amplitude * cos(pi * u / RunTime);
    else
        % Khi het thoi gian, giu nguyen vi tri tai dich
        x = End_Point;
    end
    
end

== matlab function Straight_line/Subsystem/Subsystem1/MATLAB Function1 ==
  data: u input; y output
function y = Ye_func(u)

y = 0;
end

== matlab function Straight_line/Subsystem/Subsystem1/MATLAB Function2 ==
  data: u input; z output
function z = Ze_func(u)

   %z =  ;
   %z =  -14;
   z =  -6;
end

== matlab function Straight_line/Subsystem3/Forward Kinematic ==
  data: Theta1 input; X output; Theta2 input; Theta3 input; Y output; Z output
%% -------- Forward Kinematics --------
function [X,Y,Z] = ForwardKinematics(Theta1,Theta2,Theta3)
    % Tham số đã cho
    L0 = 13; L1 = 7; L2 = 11; L3 = 7;

    T10 = [cos(Theta1), -sin(Theta1), 0, 0;
           sin(Theta1),  cos(Theta1), 0, 0;
           0,             0,          1, 0;
           0,             0,          0, 1];

    T21 = [cos(Theta2), -sin(Theta2), 0, 0;
           0,            0,           1, L1;
           -sin(Theta2), -cos(Theta2),0, 0;
           0,            0,           0, 1];

    T32 = [cos(Theta3), -sin(Theta3), 0, L2;
           sin(Theta3),  cos(Theta3), 0, 0;
           0,            0,           1, 0;
           0,            0,           0, 1];

    Te3 = [1, 0, 0, L3;
           0, 1, 0, 0;
           0, 0, 1, 0;
           0, 0, 0, 1];

    T0W = [1,0,0,0;
           0,0,1,0;
           0,-1,0,L0;
           0,0,0,1];

    T20 = T10*T21;
    T30 = T20*T32;
    Te0 = T30*Te3;
    TeW = T0W*Te0;

    X = TeW(1,4);
    Y = TeW(2,4);
    Z = TeW(3,4);
end

== matlab function Straight_line/Subsystem/Inverse Kinematic ==
  data: Xd input; Yd input; Zd input; Select_Mode input; clk input; Theta1_des output; Theta2_des output; Theta3_des output; Theta1_dot_des output; Theta2_dot_des output; Theta3_dot_des output; Theta1_ddot_des output; Theta2_ddot_des output; Theta3_ddot_des output
function [Theta1_des, Theta2_des, Theta3_des, ...
          Theta1_dot_des, Theta2_dot_des, Theta3_dot_des, ...
          Theta1_ddot_des, Theta2_ddot_des, Theta3_ddot_des] = InverseKinematics(Xd, Yd, Zd, Select_Mode, clk)
% ============================================================
% UNIFIED INVERSE KINEMATICS (Straight Line & Circle)
% Input Select_Mode:
%   1: Straight Line Trajectory
%   2: Circular Trajectory
% ============================================================

    % --- 1. THONG SO HINH HOC (CHUNG CHO CA 2) ---
    L1 = 7;
    L2 = 11;
    L3 = 7;
    L0 = 13; 

    % --- 2. TINH TOAN DAO HAM (QUY HOACH QUY DAO) ---
    % Khoi tao gia tri mac dinh
    Xd_dot = 0; Xd_ddot = 0;
    Yd_dot = 0; Yd_ddot = 0;
    Zd_dot = 0; Zd_ddot = 0;

    if Select_Mode == 1
        %% --- CHE DO 1: DUONG THANG (Straight Line) ---
        Start_Point = -2;
        End_Point = 2;
        A = (End_Point - Start_Point) / 2; % Bien do = 2
        
        TravelTime = 25;              % Thoi gian di chuyen
        w = pi / TravelTime;          % Tan so goc

        % Truc X (Cosine Trajectory)
        Xd_dot  = A * w * sin(w * clk);
        Xd_ddot = A * w^2 * cos(w * clk);
        
        % Truc Y va Z (Giữ nguyen = 0 va const)
        Yd_dot = 0; Yd_ddot = 0;
        Zd_dot = 0; Zd_ddot = 0;

    else
        %% --- CHE DO 2: HINH TRON (Circle) ---
        T = 5;                        % Chu ky
        w = 2*pi/T;                   % Tan so goc
        R = 2;                        % Ban kinh quy dao

        % Dao ham cap 1
        Xd_dot  =  R * w * cos(w*clk + pi/2);
        Yd_dot  = -R * w * sin(w*clk + pi/2);
        Zd_dot  = 0;

        % Dao ham cap 2
        Xd_ddot = -R * w^2 * sin(w*clk + pi/2);
        Yd_ddot = -R * w^2 * cos(w*clk + pi/2);
        Zd_ddot = 0;
    end

    % ============================================================
    % --- 3. GIAI BAI TOAN DONG HOC NGUOC (CORE SOLVER) ---
    % ============================================================

    % --- Buoc 3.1: Tinh Theta2, Theta3 ---
    sinTheta2 = -Yd / L2;
    
    % Rang buoc gia tri trong khoang [-1, 1] 
    sinTheta2 = min(max(sinTheta2, -1), 1);
    
    Theta2_des = asin(sinTheta2);
    Theta3_des = -Theta2_des;   % Rang buoc Elbow-up/Parallel
    
    cosTheta2 = cos(Theta2_des); % Tinh cos(Theta2)

    % --- Dao ham Theta2, Theta3 ---
    % Check Singularity (tranh chia cho 0)
    if abs(cosTheta2) < 1e-6
        Theta2_dot_des = 0;
        Theta2_ddot_des = 0;
    else
        Theta2_dot_des = -Yd_dot / (L2 * cosTheta2);
        Theta2_ddot_des = (-Yd_ddot / (L2 * cosTheta2)) - (Theta2_dot_des^2 * tan(Theta2_des));
    end

    Theta3_dot_des = -Theta2_dot_des;
    Theta3_ddot_des = -Theta2_ddot_des;

    % --- Buoc 3.2: Tinh Theta1 ---
    D = L2*cosTheta2 + L3;
    d = Zd - L0;
    
    % Cong thuc hinh hoc
    F = (-d - Xd*(L1/D));
    H = (Xd - d*(L1/D));
    Theta1_des = atan2(F, H);

    % --- Dao ham F, H ---
    D_dot = -L2*sin(Theta2_des)*Theta2_dot_des;
    D_ddot = -L2*(cos(Theta2_des)*Theta2_dot_des^2 + sin(Theta2_des)*Theta2_ddot_des);

    % Bao ve mau so D 
    if abs(D) < 1e-6; D = 1e-6; end

    F_dot = -(Zd_dot) - Xd_dot*(L1/D) + Xd*(L1*D_dot)/(D^2);
    H_dot = Xd_dot - Zd_dot*(L1/D) + d*(L1*D_dot)/(D^2);

    F_ddot = -(Zd_ddot) - Xd_ddot*(L1/D) ...
             + 2*Xd_dot*(L1*D_dot)/(D^2) ...
             - Xd*(L1*D_ddot)/(D^2) + 2*Xd*(L1*D_dot^2)/(D^3);

    H_ddot = Xd_ddot - Zd_ddot*(L1/D) ...
             + 2*Zd_dot*(L1*D_dot)/(D^2) ...
             - d*(L1*D_ddot)/(D^2) + 2*d*(L1*D_dot^2)/(D^3);

    % --- Dao ham Theta1 ---
    denominator = F^2 + H^2;
    
    % Check Singularity cho mau so cua Theta1
    if denominator < 1e-6
        Theta1_dot_des = 0;
        Theta1_ddot_des = 0;
    else
        Theta1_dot_des = (H*F_dot - F*H_dot) / denominator;
        Theta1_ddot_des = ((H*F_ddot - F*H_ddot)*denominator ...
                          - 2*(H*F_dot - F*H_dot)*(F*F_dot + H*H_dot)) ...
                          / (denominator^2);
    end
end

== matlab function Straight_line/Subsystem/Subsystem/MATLAB Function ==
  data: u input; x output
function x = Xe_func(u)
% Xe_func: Tính tọa độ X của quỹ đạo đường tròn
% Input:
%   u - thời gian (hoặc biến độc lập từ Clock)
% Output:
%   y - giá trị Xe

    R = 2;   % bán kính
    x = R * sin((2*pi/5)*u + pi/2);
end

== matlab function Straight_line/Subsystem/Subsystem/MATLAB Function1 ==
  data: u input; y output
function y = Ye_func(u)
% Ye_func: Tính tọa độ Y của quỹ đạo đường tròn
% Input:
%   u - thời gian (hoặc biến độc lập từ Clock)
% Output:
%   y - giá trị Ye

    R = 2;   % bán kính
    y = R * cos((2*pi/5)*u + pi/2);
end

== matlab function Straight_line/Subsystem1/Torque Compute/Computed Torque ==
  data: Theta1 input; Torque1 output; Theta2 input; Theta3 input; Theta1_dot input; Theta2_dot input; Theta3_dot input; Theta1_des input; Theta2_des input; Theta3_des input; Theta1_dot_des input; Theta2_dot_des input; Theta3_dot_des input; Theta1_ddot_des input; Theta2_ddot_des input; Theta3_ddot_des input; Torque2 output; Torque3 output
function [Torque1, Torque2, Torque3] = ComputedTorqueController3DOF( ...
    Theta1, Theta2, Theta3, ...
    Theta1_dot, Theta2_dot, Theta3_dot, ...
    Theta1_des, Theta2_des, Theta3_des, ...
    Theta1_dot_des, Theta2_dot_des, Theta3_dot_des, ...
    Theta1_ddot_des, Theta2_ddot_des, Theta3_ddot_des)

%% ---------------- Parameters ----------------
L1 = 7; 
L2 = 11;
L3 = 7;

m1 = 79168.13487; 
m2 = 29700; 
m3 = 6300;

I1 = 402437.875; 
I2 = 1197900; 
I3 = 102900;

lc1 = L1 / 2;
lc2 = L2 / 2;
lc3 = L3 / 2;

g = 9.81;

%% ---------------- Desired and actual vectors ----------------
Theta     = [Theta1; Theta2; Theta3];
Theta_dot = [Theta1_dot; Theta2_dot; Theta3_dot];
Theta_des = [Theta1_des; Theta2_des; Theta3_des];
Theta_dot_des = [Theta1_dot_des; Theta2_dot_des; Theta3_dot_des];
Theta_ddot_des = [Theta1_ddot_des; Theta2_ddot_des; Theta3_ddot_des];

%% ---------------- Error terms ----------------
E     = Theta_des - Theta;
E_dot = Theta_dot_des - Theta_dot;

%% ---------------- Dynamic model ----------------
% --- Inertia matrix M(Theta)
M11 = I1 + I2 + I3 ...
    + m1*lc1^2 ...
    + m2*(L1^2 + lc2^2 + 2*L1*lc2*cos(Theta2)) ...
    + m3*(L1^2 + L2^2 + lc3^2 ...
          + 2*L1*L2*cos(Theta2) ...
          + 2*L1*lc3*cos(Theta2 + Theta3) ...
          + 2*L2*lc3*cos(Theta3));

M12 = I2 + I3 ...
    + m2*(lc2^2 + L1*lc2*cos(Theta2)) ...
    + m3*(L2^2 + lc3^2 + L1*L2*cos(Theta2) ...
          + L1*lc3*cos(Theta2 + Theta3) ...
          + L2*lc3*cos(Theta3));

M13 = I3 + m3*(lc3^2 + L1*lc3*cos(Theta2 + Theta3) + L2*lc3*cos(Theta3));

M22 = I2 + I3 ...
    + m2*lc2^2 ...
    + m3*(L2^2 + lc3^2 + 2*L2*lc3*cos(Theta3));

M23 = I3 + m3*(lc3^2 + L2*lc3*cos(Theta3));

M33 = I3 + m3*lc3^2;

M = [M11, M12, M13;
     M12, M22, M23;
     M13, M23, M33];

% --- Coriolis/Centrifugal matrix C(Theta, Theta_dot)
h1 = -m2*L1*lc2*sin(Theta2) ...
     - m3*L1*L2*sin(Theta2) ...
     - m3*L1*lc3*sin(Theta2 + Theta3);
h2 = -m3*L2*lc3*sin(Theta3);

C = [ h1*(Theta2_dot + Theta3_dot),  h1*(Theta2_dot + Theta3_dot),  h1*Theta3_dot;
     -h1*Theta1_dot,                 h2*Theta3_dot,                 h2*(Theta2_dot + Theta3_dot);
     -h1*Theta1_dot,                -h2*(Theta1_dot + Theta2_dot),  0];

% --- Gravity vector G(Theta)
G1 = (m1*lc1 + m2*L1 + m3*L1)*g*cos(Theta1) ...
   + (m2*lc2 + m3*L2)*g*cos(Theta1 + Theta2) ...
   + m3*lc3*g*cos(Theta1 + Theta2 + Theta3);

G2 = (m2*lc2 + m3*L2)*g*cos(Theta1 + Theta2) ...
   + m3*lc3*g*cos(Theta1 + Theta2 + Theta3);

G3 = m3*lc3*g*cos(Theta1 + Theta2 + Theta3);

G = [G1; G2; G3];

%% ---------------- Controller gains ----------------

Kp = diag([1800, 5400, 450]);   % bộ Kp, Kd với hình tròn   
Kd = diag([180, 540, 45]);

%Kp = diag([3200, 9600, 800]);   % Bộ Kp, Kd với đường thẳng   
%Kd = diag([320, 960, 80]);

%% ---------------- Computed Torque ----------------
Torque = M*(Theta_ddot_des + Kd*E_dot + Kp*E) + C*Theta_dot + G;

%% ---------------- Outputs ----------------
Torque1 = Torque(1);
Torque2 = Torque(2);
Torque3 = Torque(3);

end
